simulink library "act"  (Simulink 8.1)
settings: Solver=ode45  StartTime=0.0  StopTime=10.0  RelTol=1e-3
undefined symbols (not defined in the file or in its folder): C_TICK_TIME_S, FALSE, KIFO_ActiveDriverTimer_ms, KIFO_SWSActiveDriver_degps, KIFO_ThrottlePosTimeDelay_ms, KIFO_ThrottleVariationAct_pctps, TRUE
libraries: hcu_lib x2, idiada_lib x1
settings Model: Creator=xsellart  LastModifiedBy=tescamilla

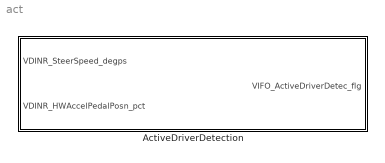
== system act ==
  ActiveDriverDetection : Subsystem

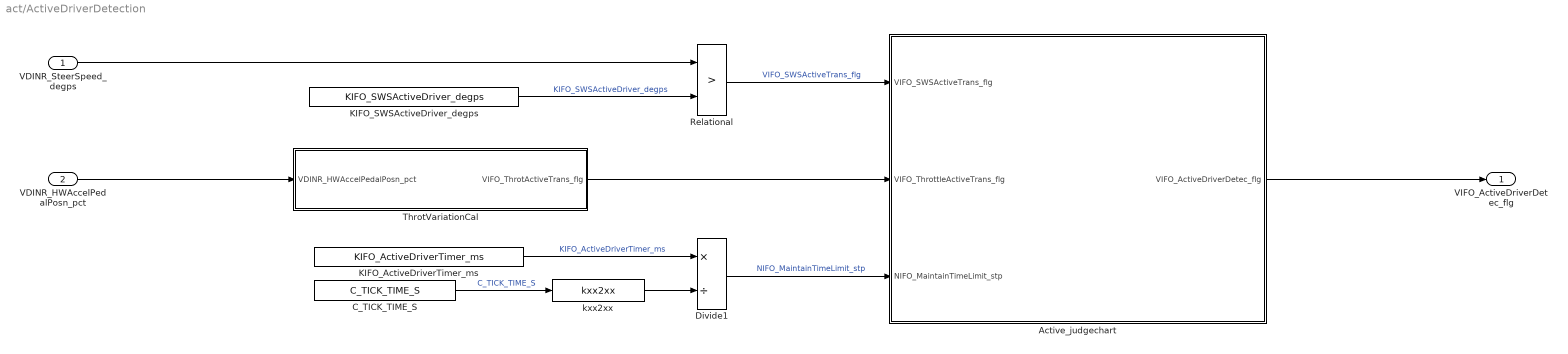
== system act/ActiveDriverDetection ==
  VDINR_SteerSpeed_degps : Inport
  VDINR_HWAccelPedalPosn_pct : Inport  Port=2
  Active_judgechart : Stateflow chart  TreatAsAtomicUnit=on
  C_TICK_TIME_S : Constant  Value=C_TICK_TIME_S
  Divide1 : Product  Inputs=*/
  KIFO_ActiveDriverTimer_ms : Constant  Value=KIFO_ActiveDriverTimer_ms  OutDataTypeStr=single
  KIFO_SWSActiveDriver_degps : Constant  Value=KIFO_SWSActiveDriver_degps
  Relational : RelationalOperator  Operator=>  OutDataTypeStr=boolean
  ThrotVariationCal : Subsystem
  kxx2xx : hcu_lib/kxx2xx
  VIFO_ActiveDriverDetec_flg : Outport
  wires:
  ThrotVariationCal/1(VIFO_ThrotActiveTrans_flg) -> Active_judgechart/2(VIFO_ThrottleActiveTrans_flg)
  VDINR_HWAccelPedalPosn_pct/1 -> ThrotVariationCal/1(VDINR_HWAccelPedalPosn_pct)
  C_TICK_TIME_S/1 -> kxx2xx/1  "C_TICK_TIME_S"
  Divide1/1 -> Active_judgechart/3(NIFO_MaintainTimeLimit_stp)  "NIFO_MaintainTimeLimit_stp"
  kxx2xx/1 -> Divide1/2
  KIFO_ActiveDriverTimer_ms/1 -> Divide1/1  "KIFO_ActiveDriverTimer_ms"
  Relational/1 -> Active_judgechart/1(VIFO_SWSActiveTrans_flg)  "VIFO_SWSActiveTrans_flg"
  Active_judgechart/1(VIFO_ActiveDriverDetec_flg) -> VIFO_ActiveDriverDetec_flg/1
  KIFO_SWSActiveDriver_degps/1 -> Relational/2  "KIFO_SWSActiveDriver_degps"
  VDINR_SteerSpeed_degps/1 -> Relational/1

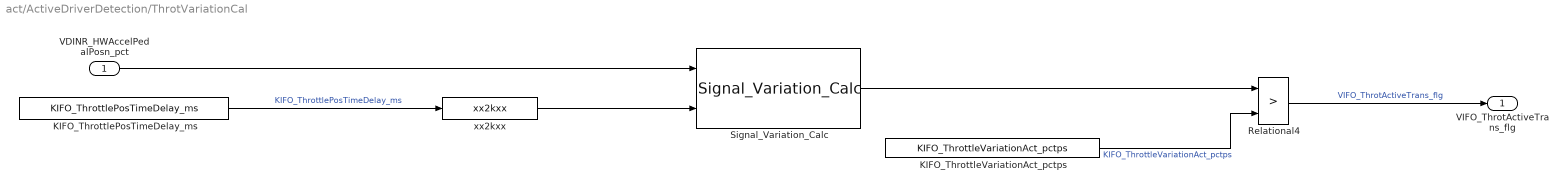
== system act/ActiveDriverDetection/ThrotVariationCal ==
  VDINR_HWAccelPedalPosn_pct : Inport
  KIFO_ThrottlePosTimeDelay_ms : Constant  Value=KIFO_ThrottlePosTimeDelay_ms
  KIFO_ThrottleVariationAct_pctps : Constant  Value=KIFO_ThrottleVariationAct_pctps  OutDataTypeStr=single
  Relational4 : RelationalOperator  Operator=>  OutDataTypeStr=boolean
  Signal_Variation_Calc : idiada_lib/Signal_Variation_Calc
  xx2kxx : hcu_lib/xx2kxx
  VIFO_ThrotActiveTrans_flg : Outport
  wires:
  xx2kxx/1 -> Signal_Variation_Calc/2
  Relational4/1 -> VIFO_ThrotActiveTrans_flg/1  "VIFO_ThrotActiveTrans_flg"
  Signal_Variation_Calc/1 -> Relational4/1
  KIFO_ThrottleVariationAct_pctps/1 -> Relational4/2  "KIFO_ThrottleVariationAct_pctps"
  KIFO_ThrottlePosTimeDelay_ms/1 -> xx2kxx/1  "KIFO_ThrottlePosTimeDelay_ms"
  VDINR_HWAccelPedalPosn_pct/1 -> Signal_Variation_Calc/1

== stateflow chart ActiveDriverDetection/Active_judgechart ==
  state OFF
    en:
    VIFO_ActiveDriverDetec_flg = FALSE;
  state ON
    en:
    VIFO_ActiveDriverDetec_flg = TRUE;
  state MAINTAIN
    en:
    NIFO_MaintainTimeLocal_stp = 0;
    du:
    NIFO_MaintainTimeLocal_stp =NIFO_MaintainTimeLocal_stp+1;
  (default) -> OFF
  (junction 13) -> OFF : [NIFO_MaintainTimeLocal_stp > NIFO_MaintainTimeLimit_stp]
  MAINTAIN -> (junction 13) [order 2]
  OFF -> (junction 14)
  MAINTAIN -> ON [order 1] : [VIFO_SWSActiveTrans_flg==TRUE ...
      | || VIFO_ThrottleActiveTrans_flg==TRUE]
  (junction 14) -> ON : [VIFO_SWSActiveTrans_flg==TRUE ...
      | || VIFO_ThrottleActiveTrans_flg==TRUE]
  ON -> MAINTAIN : [VIFO_SWSActiveTrans_flg==FALSE ...
      | && VIFO_ThrottleActiveTrans_flg==FALSE]
  data: VIFO_ActiveDriverDetec_flg output boolean; VIFO_SWSActiveTrans_flg input boolean; VIFO_ThrottleActiveTrans_flg input boolean; TRUE parameter double; FALSE parameter double; NIFO_MaintainTimeLocal_stp local single; NIFO_MaintainTimeLimit_stp input single
